simulink subsystem "sensors"  (R2022a)
settings: Solver=VariableStepAuto  StartTime=0.0  StopTime=10.0  RelTol=1e-3
model mask{rg=1e-10, rtg=1e-10, ra=1e-10, rm=1e-10, B0=0, dt=0.01}
  mask prompts: rg "Gyroscope RMS noise [rad/s]"; rtg "Gyroscope RMS drift [rad/s^2]"; ra "Accelerometer RMS noise [m/s^2]"; rm "Magnetometer RMS noise [gauss]"; B0 "Reference magnetic field [gauss]"; dt "Sample time [s]"
libraries: sm_lib x3, nesl_utility x1
settings Model: Creator=yevge  LastModifiedBy=yevge

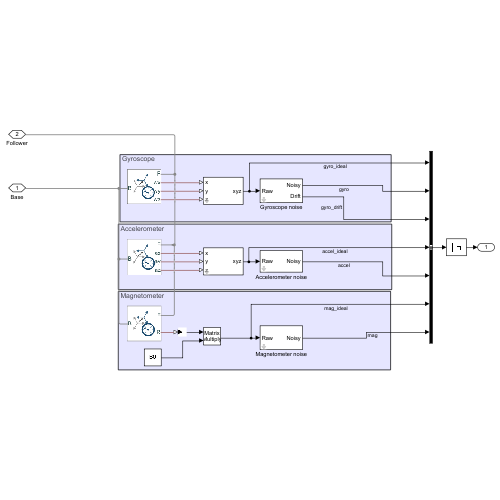
[thumbnail: Simulink's stored preview of the top-level diagram]
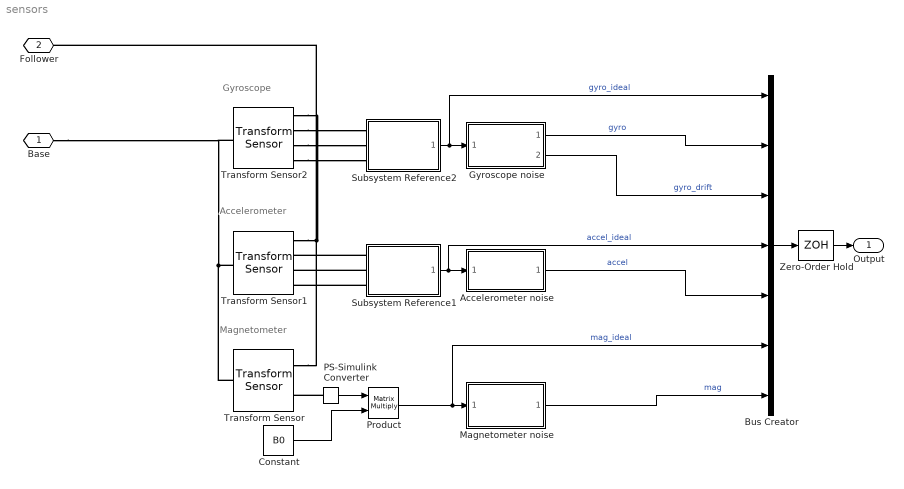
== system sensors ==
  note: Magnetometer
  note: Accelerometer
  note: Gyroscope
  Accelerometer noise : Subsystem  ReferencedSubsystem=additive_unbiased_sensor  r=ra  dt=dt
  Bus Creator : BusCreator  Inputs=7
  Constant : Constant  Value=B0
  Gyroscope noise : Subsystem  ReferencedSubsystem=additive_biased_sensor  r=rg  rt=rtg  dt=dt
  Magnetometer noise : Subsystem  ReferencedSubsystem=additive_unbiased_sensor  r=rm  dt=dt
  PS-Simulink Converter : nesl_utility/PS-Simulink Converter  PhysicalDomain=network_engine_domain  SubClassName=ps_output  LeftPortType=input  RightPortType=output  PseudoPeriodic=off  Frequencies=[]  VectorFormat=inherit  Unit=inherit  AffineConversion=off
      settings: SourceProductBaseCode=SS,PW,VE
  Product : Product  Multiplication=Matrix(*)
  Subsystem Reference1 : Subsystem  ReferencedSubsystem=PS_Simulink_3x  Unit=m/s^2
  Subsystem Reference2 : Subsystem  ReferencedSubsystem=PS_Simulink_3x  Unit=rad/s
  Transform Sensor : sm_lib/Frames and Transforms/Transform Sensor  MeasurementFrame=World  SenseAngle=off  SenseAxis=off  SenseAngle1=off  SenseAngle2=off  SenseAngle3=off  SenseQ=off  SenseR=on  SenseOmegaX=off  SenseOmegaY=off  SenseOmegaZ=off  SenseOmega1=off  SenseOmega2=off  SenseOmega3=off  SenseQDot=off  SenseRDot=off  SenseAlphaX=off  SenseAlphaY=off  SenseAlphaZ=off  SenseAlpha1=off  SenseAlpha2=off  SenseAlpha3=off  SenseQDDot=off  SenseRDDot=off  SenseX=off  SenseY=off  SenseZ=off  SenseRad=off  SenseAzim=off  SenseDist=off  SenseInc=off  SenseXDot=off  SenseYDot=off  SenseZDot=off  SenseRadDot=off  SenseAzimDot=off  SenseDistDot=off  SenseIncDot=off  SenseXDDot=off  SenseYDDot=off  SenseZDDot=off  SenseRadDDot=off  SenseAzimDDot=off  SenseDistDDot=off  SenseIncDDot=off
  Transform Sensor1 : sm_lib/Frames and Transforms/Transform Sensor  MeasurementFrame=NonRotatingFollower  SenseAngle=off  SenseAxis=off  SenseAngle1=off  SenseAngle2=off  SenseAngle3=off  SenseQ=off  SenseR=off  SenseOmegaX=off  SenseOmegaY=off  SenseOmegaZ=off  SenseOmega1=off  SenseOmega2=off  SenseOmega3=off  SenseQDot=off  SenseRDot=off  SenseAlphaX=off  SenseAlphaY=off  SenseAlphaZ=off  SenseAlpha1=off  SenseAlpha2=off  SenseAlpha3=off  SenseQDDot=off  SenseRDDot=off  SenseX=off  SenseY=off  SenseZ=off  SenseRad=off  SenseAzim=off  SenseDist=off  SenseInc=off  SenseXDot=off  SenseYDot=off  SenseZDot=off  SenseRadDot=off  SenseAzimDot=off  SenseDistDot=off  SenseIncDot=off  SenseXDDot=on  SenseYDDot=on  SenseZDDot=on  SenseRadDDot=off  SenseAzimDDot=off  SenseDistDDot=off  SenseIncDDot=off
  Transform Sensor2 : sm_lib/Frames and Transforms/Transform Sensor  MeasurementFrame=Follower  SenseAngle=off  SenseAxis=off  SenseAngle1=off  SenseAngle2=off  SenseAngle3=off  SenseQ=off  SenseR=off  SenseOmegaX=on  SenseOmegaY=on  SenseOmegaZ=on  SenseOmega1=off  SenseOmega2=off  SenseOmega3=off  SenseQDot=off  SenseRDot=off  SenseAlphaX=off  SenseAlphaY=off  SenseAlphaZ=off  SenseAlpha1=off  SenseAlpha2=off  SenseAlpha3=off  SenseQDDot=off  SenseRDDot=off  SenseX=off  SenseY=off  SenseZ=off  SenseRad=off  SenseAzim=off  SenseDist=off  SenseInc=off  SenseXDot=off  SenseYDot=off  SenseZDot=off  SenseRadDot=off  SenseAzimDot=off  SenseDistDot=off  SenseIncDot=off  SenseXDDot=off  SenseYDDot=off  SenseZDDot=off  SenseRadDDot=off  SenseAzimDDot=off  SenseDistDDot=off  SenseIncDDot=off
  Zero-Order Hold : ZeroOrderHold  SampleTime=dt
  Base : PMIOPort  Side=Left
  Follower : PMIOPort  Port=2  Side=Left
  Output : Outport
  wires:
  Accelerometer noise/1 -> Bus Creator/5  "accel"
  PS-Simulink Converter/1 -> Product/1
  Product/1 -> Bus Creator/6, Magnetometer noise/1  "mag_ideal"
  Magnetometer noise/1 -> Bus Creator/7  "mag"
  Subsystem Reference1/1 -> Bus Creator/4, Accelerometer noise/1  "accel_ideal"
  Subsystem Reference2/1 -> Bus Creator/1, Gyroscope noise/1  "gyro_ideal"
  Bus Creator/1 -> Zero-Order Hold/1
  Gyroscope noise/1 -> Bus Creator/2  "gyro"
  Gyroscope noise/2 -> Bus Creator/3  "gyro_drift"
  Constant/1 -> Product/2
  Zero-Order Hold/1 -> Output/1
  connections:
  Transform Sensor1/LConn1 -- Base/RConn1 -- Transform Sensor2/LConn1 -- Transform Sensor/LConn1
  Transform Sensor/RConn1 -- Follower/RConn1 -- Transform Sensor2/RConn1 -- Transform Sensor1/RConn1
  PS-Simulink Converter/LConn1 -- Transform Sensor/RConn2
  Subsystem Reference1/LConn1 -- Transform Sensor1/RConn2
  Subsystem Reference1/LConn3 -- Transform Sensor1/RConn4
  Subsystem Reference1/LConn2 -- Transform Sensor1/RConn3
  Transform Sensor2/RConn4 -- Subsystem Reference2/LConn3
  Transform Sensor2/RConn3 -- Subsystem Reference2/LConn2
  Transform Sensor2/RConn2 -- Subsystem Reference2/LConn1
